simulink model "ejemplo6"  (R2020b)
settings: Solver=VariableStepAuto  StartTime=0.0  StopTime=1  MaxStep=1e-3  RelTol=1e-3
values from neighbouring files (symbols this model uses):
  p0 = x(4)    [ejemplo_6.m]
  p01 = x(6)    [ejemplo_6.m]
  p1 = x(3)    [ejemplo_6.m]
  p11 = x(5)    [ejemplo_6.m]
  p21 = x(4)    [ejemplo_6.m]
  q0 = x(2)    [ejemplo_6.m]
  q01 = x(3)    [ejemplo_6.m]
  q1 = x(1)    [ejemplo_6.m]
  q11 = x(2)    [ejemplo_6.m]
  q21 = x(1)    [ejemplo_6.m]
libraries: pid_lib x1
settings Model: Creator=carma  LastModifiedBy=Acer

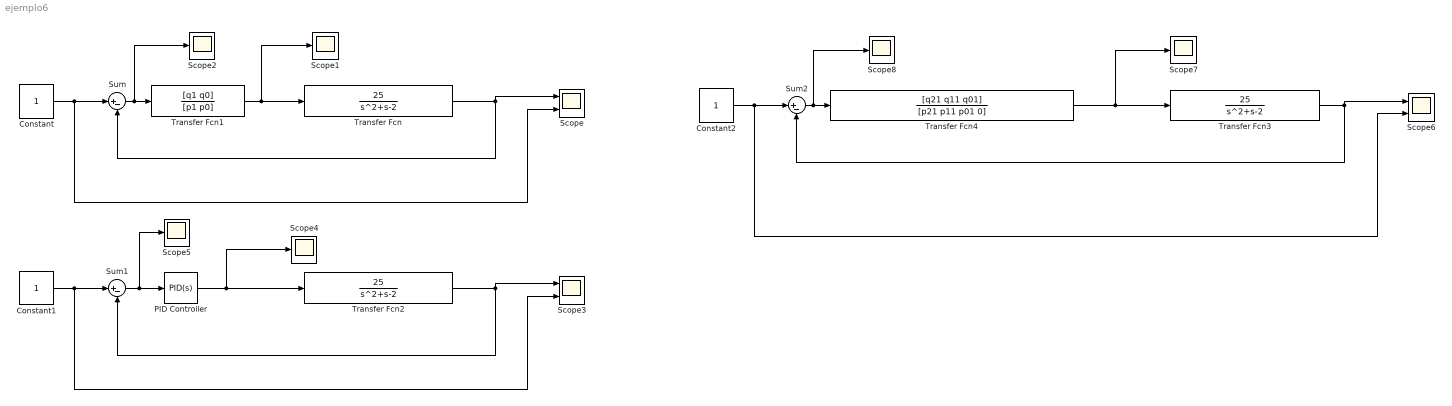
== system ejemplo6 ==
  Constant : Constant  VectorParams1D=off  SampleTime=-1
  Constant1 : Constant  VectorParams1D=off  SampleTime=-1
  Constant2 : Constant  VectorParams1D=off  SampleTime=-1
  PID Controller : pid_lib/PID Controller  Controller=PID  Form=Parallel  TimeDomain=Continuous-time  UseExternalTs=off  SampleTime=-1  IntegratorMethod=Forward Euler  FilterMethod=Forward Euler  ControllerParametersSource=internal  P=28.1436486179847  I=84.6444415395738  D=2.28714534896611  UseFilter=on  N=321.534636328263  TunerSelectOption=Transfer Function Based (PID Tuner App)  InitialConditionSource=internal  InitialConditionForIntegrator=0  InitialConditionForFilter=0  DifferentiatorICPrevScaledInput=0  ExternalReset=none  TrackingMode=off  Kt=1  LimitOutput=off  SatLimitsSource=internal  UpperSaturationLimit=inf  LowerSaturationLimit=-inf  LinearizeAsGain=on  AntiWindupMode=none  Kb=1  POutMin=[]  POutMax=[]  IOutMin=[]  IOutMax=[]  DOutMin=[]  DOutMax=[]  NOutMin=[]  NOutMax=[]  SumOutMin=[]  SumOutMax=[]  SaturationOutMin=[]  SaturationOutMax=[]  PParamMin=[]  PParamMax=[]  IParamMin=[]  IParamMax=[]  DParamMin=[]  DParamMax=[]  NParamMin=[]  NParamMax=[]  KbParamMin=[]  KbParamMax=[]  KtParamMin=[]  KtParamMax=[]  KbOutMin=[]  KbOutMax=[]  KtOutMin=[]  KtOutMax=[]  IntegratorOutMin=[]  IntegratorOutMax=[]  FilterOutMin=[]  FilterOutMax=[]  SumI1OutMin=[]  SumI1OutMax=[]  SumI2OutMin=[]  SumI2OutMax=[]  SumI3OutMin=[]  SumI3OutMax=[]  SumI4OutMin=[]  SumI4OutMax=[]  SumDOutMin=[]  SumDOutMax=[]  DifferentiatorOutMin=[]  DifferentiatorOutMax=[]  FilterDiffOutCoefMin=[]  FilterDiffOutCoefMax=[]  ReciprocalOutMin=[]  ReciprocalOutMax=[]  SumDenOutMin=[]  SumDenOutMax=[]  SumNumOutMin=[]  SumNumOutMax=[]  DivideOutMin=[]  DivideOutMax=[]  UdiffTsProdOutMin=[]  UdiffTsProdOutMax=[]  NTsProdOutMin=[]  NTsProdOutMax=[]  UintegralTsProdOutMin=[]  UintegralTsProdOutMax=[]  UngainTsProdOutMin=[]  UngainTsProdOutMax=[]  IntegratorContinuousStateAttributes=''  IntegratorStateMustResolveToSignalObject=off  IntegratorRTWStateStorageClass=Auto  FilterContinuousStateAttributes=''  FilterStateMustResolveToSignalObject=off  FilterRTWStateStorageClass=Auto  ParallelPVariant=InternalParameters  IdealPVariant=Disabled  IVariant=InternalParameters  DVariant=InternalParameters  IntegratorVariant=Continuous  SatVariant=Disabled  AWVariant=Passthrough  PCopyVariant=Disabled  TRVariant=Disabled  FdbkBlocksVariant=Forward  IdealPFdbkVariant=Disabled  SatFdbkVariant=Disabled  DerivativeFilterVariant=ContFilter  NVariant=InternalParameters  NCopyVariant=Disabled  FilterICVariant=InternalICsFilter  IntegratorICVariant=InternalICs  ExternalResetVariant=Disabled  TRSumVariant=Passthrough  SumFdbkVariant=Disabled  SumVariant=Sum_PID  TsampFilterVariant=InternalTs  TsampNgainVariant=Passthrough  TsampIntegralVariant=Passthrough  ExternalSaturationOutDataTypeStr=Inherit: Same as second input
  Scope : Scope  NumInputPorts=2
  Scope{1..2,4..5,7..8} (6 alike) : Scope
  Scope3 : Scope  NumInputPorts=2
  Scope6 : Scope  NumInputPorts=2
  Sum : Sum  Inputs=|+-
  Sum1 : Sum  Inputs=|+-
  Sum2 : Sum  Inputs=|+-
  Transfer Fcn : TransferFcn  Numerator=[25]  Denominator=[1 1 -2]
  Transfer Fcn1 : TransferFcn  Numerator=[q1 q0]  Denominator=[p1 p0]
  Transfer Fcn2 : TransferFcn  Numerator=[25]  Denominator=[1 1 -2]
  Transfer Fcn3 : TransferFcn  Numerator=[25]  Denominator=[1 1 -2]
  Transfer Fcn4 : TransferFcn  Numerator=[q21 q11 q01]  Denominator=[p21 p11 p01 0]
  wires:
  Transfer Fcn1/1 -> Transfer Fcn/1, Scope1/1
  Sum/1 -> Scope2/1, Transfer Fcn1/1
  Transfer Fcn/1 -> Scope/1, Sum/2
  Constant/1 -> Scope/2, Sum/1
  Constant1/1 -> Scope3/2, Sum1/1
  Sum1/1 -> PID Controller/1, Scope5/1
  Transfer Fcn2/1 -> Scope3/1, Sum1/2
  PID Controller/1 -> Transfer Fcn2/1, Scope4/1
  Sum2/1 -> Scope8/1, Transfer Fcn4/1
  Transfer Fcn3/1 -> Scope6/1, Sum2/2
  Constant2/1 -> Scope6/2, Sum2/1
  Transfer Fcn4/1 -> Scope7/1, Transfer Fcn3/1
